simulink model "tqdtqr_rebuild_V3"  (R2021b)
settings: Solver=VariableStepAuto  StartTime=0.0  StopTime=10.0  RelTol=1e-3
undefined symbols (not defined in the file): ATQD_AfterTqMinGain_X_Deg, ATQD_APSCreepBaseTqD_X_kph, ATQD_APSCreepBaseTqD_Y_Deg, ATQD_APSCreepBaseTqR_X_kph, ATQD_APSCreepBaseTqR_Y_Deg, ATQD_APSCreepIterm_X_kph, ATQD_APSCreepIterm_Y_kph, ATQD_APSCreepPterm_X_kph, ATQD_APSCreepPterm_Y_kph, ATQD_APSDecReq_X_kph, ATQD_APSDecReq_Y_mps2, ATQD_APSDecReqCMD_X_kph, ATQD_APSDecReqTs_X_pct, ATQD_APSDecTimeGain_X_Deg, ATQD_APSDecTimeGain_Y_s, ATQD_APSReqLowSpd_X_Deg, ATQD_AutoHoldReleaseBPS_X_Deg, ATQD_AWDLoadTrqnsGain_X_kg, ATQD_AWDLoadTrqnsGain_Y_pct, ATQD_BOSEnBPSPosn_X_kph, ATQD_BOSMap_X_rpm, ATQD_BOSMap_Y_pct, ATQD_CreepBaseTqD_X_kph, ATQD_CreepBaseTqD_Y_Deg, ATQD_CreepBaseTqR_X_kph, ATQD_CreepBaseTqR_Y_Deg, ATQD_CreepBPSDisPosn_X_Deg, ATQD_CreepBPSDisPosnR_X_Deg, ATQD_CreepBPSEnPosn_X_Deg, ATQD_CreepBPSEnPosnR_X_Deg, ATQD_CreepDeltaTq_X_kph, ATQD_CreepIterm_X_kph, ATQD_CreepIterm_Y_kph, ATQD_CreepItermMaxLimit_X_pct, ATQD_CreepPreloadTime_X_kph, ATQD_CreepPreloadTq_X_kph, ATQD_CreepPreloadTq_Y_s, ATQD_CreepProtTq_X_Deg, ATQD_CreepPterm_X_kph, ATQD_CreepPterm_Y_kph, ATQD_CreepRrTqSpRat_X_rpm, ATQD_CreepRrTqSpRat_Y_Nm, ATQD_CreepTargetSpdD_X_pct, ATQD_CreepTargetSpdR_X_pct, ATQD_CreepUpLimitTq_X_rpm, ATQD_DecIneOPDHoldEnDelay_X_Deg, ATQD_DecIneOPDHoldEnDelay_Y_bar, ATQD_ECOTqMapD_X_rpm, ATQD_ECOTqMapD_Y_pct, ATQD_EMTqMapD_X_rpm, ATQD_EMTqMapD_Y_pct, ATQD_EOPDTqMapDCon_X_rpm, ATQD_EOPDTqMapDCon_Y_Deg, ATQD_EstInitVehWeight_X_c, ATQD_FAfterTqCMDGain_X_rpm, ATQD_FAfterTqCMDGain_Y_pct, ATQD_ForceLowSpd_X_Deg, ATQD_ForcePLimitSpd_X_Deg, ATQD_FrLossMAPLowV_X_rpm, ATQD_FrLossMAPLowV_Y_Nm ... (+949)
libraries: simulink x235, hcu_lib x208, tqr x63, tqd x6
(part 6 of 37)

== system tqdtqr_rebuild_V3/Output_Convert/CrashDetect ==
  BSCPIn_outputs : Inport
  Add1 : Sum
  Add2 : Sum
  Add3 : Sum
  Bus Selector : BusSelector  OutputSignals=VPMM_PowerSta_enum,VINP_CrashSignalGPIO_flg,VINP_CrashOutputSts_enum,task_time_s,VINP_FlashCrashDetd_flg,VINP_FlashCrashUnlockReq_flg,VBCM_CTDCtrl_enum,VBCM_CrashUnlkSuccess_flg
  Constant : Constant  Value=TRUE
  Constant1 : Constant  Value=ENUM_POWERSTA_ON
  Constant{3,8,10,19,23,36} (6 alike) : Constant  Value=KTQD_CrashPWMCnt_cnt
  Constant{6,11,20,26,31,34} (6 alike) : Constant  Value=ZERO_INT
  Constant12 : Constant  Value=KTQD_50MS_cnt
  Constant13 : Constant  Value=KTQD_PwrStaTimerforCrash_s
  Constant14 : Constant  Value=ENUM_CRASHSTATE_NOCRASH
  Constant15 : Constant  Value=KTQD_DiagHCrashTimer_s
  Constant16 : Constant  Value=ENUM_CRASHSTATE_NOCRASH
  Constant17 : Constant  Value=ENUM_CRASHSTATE_NOCRASH
  Constant18 : Constant  Value=KTQD_PwrStaTimerforCrash_s
  Constant2 : Constant  Value=ENUM_POWERSTA_READY
  Constant21 : Constant  Value=KTQD_50MS_cnt
  Constant22 : Constant  Value=ZERO_FLOAT
  Constant24 : Constant  Value=KTQD_NoDiagHCrashTimer_s
  Constant25 : Constant  Value=KTQD_DiagHCrashTimer_s
  Constant27 : Constant  Value=KTQD_190MS_cnt
  Constant28 : Constant  Value=KTQD_30MS_cnt
  Constant29 : Constant  Value=KTQD_50MS_cnt
  Constant30 : Constant  Value=KTQD_210MS_cnt
  Constant32 : Constant  Value=KTQD_NoDiagHCrashTimer_s
  Constant33 : Constant  Value=KTQD_PwrDownTimerforCrash_s
  Constant35 : Constant  Value=KTQD_210MS_cnt
  Constant37 : Constant  Value=KTQD_PwrDownTimerforCrash_s
  Constant38 : Constant  Value=TRUE
  Constant39 : Constant  Value=ENUM_CTDCTRL_UNLOCKALL
  Constant4 : Constant  Value=ONE_INT
  Constant{9,40..42} (4 alike) : Constant  Value=FALSE
  Constant43 : Constant  Value=KTQD_CrashDetdHoldTime_s
  Constant5 : Constant  Value=ENUM_POWERSTA_OFF
  Constant7 : Constant  Value=KTQD_210MS_cnt
  Data Type Conversion1 : DataTypeConversion
  Data Type Conversion2 : DataTypeConversion
  Detect Change : simulink/Logic and Bit Operations/Detect Change  vinit=0  OutDataTypeStr=boolean
  Detect Increase : simulink/Logic and Bit Operations/Detect Increase  vinit=0.0  OutDataTypeStr=boolean
  Equal : RelationalOperator  Operator=~=  OutDataTypeStr=boolean  RndMeth=Simplest
  Equal{1..2,6,10} (4 alike) : RelationalOperator  Operator===  OutDataTypeStr=boolean  RndMeth=Simplest
  Equal{3,7,9,11,13..14} (6 alike) : RelationalOperator  OutDataTypeStr=boolean  RndMeth=Simplest
  Equal12 : RelationalOperator  Operator=<  OutDataTypeStr=boolean  RndMeth=Simplest
  Equal4 : RelationalOperator  Operator=~=  OutDataTypeStr=boolean  RndMeth=Simplest
  Equal5 : RelationalOperator  Operator=<  OutDataTypeStr=boolean  RndMeth=Simplest
  Equal8 : RelationalOperator  Operator=~=  OutDataTypeStr=boolean  RndMeth=Simplest
  Hold : hcu_lib/Basic_Blocks/Hold  SystemSampleTime=-1  VariantActivationTime=update diagram  Latency=0  AutoFrameSizeCalculation=off
  Latch : hcu_lib/Basic_Blocks/Latch
  Latch2 : hcu_lib/Basic_Blocks/Latch
  Logical Operator{,9..10,13,16,21,23,26} (8 alike) : Logic  Operator=OR  AllPortsSameDT=off  OutDataTypeStr=boolean
  Logical Operator{1,3,7..8,18,20} (6 alike) : Logic  Operator=NOT  AllPortsSameDT=off  OutDataTypeStr=boolean
  Logical Operator{4..5,11..12,14..15,17,19,22} (9 alike) : Logic  AllPortsSameDT=off  OutDataTypeStr=boolean
  Logical Operator2 : Logic  Inputs=3  AllPortsSameDT=off  OutDataTypeStr=boolean
  Logical Operator6 : Logic  Inputs=3  AllPortsSameDT=off  OutDataTypeStr=boolean
  Relational Operator{,5..7,9} (5 alike) : RelationalOperator  Operator=>  OutDataTypeStr=boolean  RndMeth=Simplest
  Relational Operator1 : RelationalOperator  OutDataTypeStr=boolean  RndMeth=Simplest
  Relational Operator10 : RelationalOperator  Operator=<  OutDataTypeStr=boolean  RndMeth=Simplest
  Relational Operator2 : RelationalOperator  Operator=<=  OutDataTypeStr=boolean  RndMeth=Simplest
  Relational Operator3 : RelationalOperator  OutDataTypeStr=boolean  RndMeth=Simplest
  Relational Operator4 : RelationalOperator  Operator=<=  OutDataTypeStr=boolean  RndMeth=Simplest
  Relational Operator8 : RelationalOperator  Operator=<  OutDataTypeStr=boolean  RndMeth=Simplest
  SR_Latch : hcu_lib/Basic_Blocks/SR_Latch
  SR_Latch1 : hcu_lib/Basic_Blocks/SR_Latch
  Switch{,1,10..14} (7 alike) : Switch  Criteria=u2 ~= 0
  Switch{2..9} (8 alike) : Switch  Criteria=u2 > Threshold
  Timer{1..4} (4 alike) : hcu_lib/Basic_Blocks/Timer
  Unit Delay{,1..7} (8 alike) : UnitDelay  SampleTime=-1  HasFrameUpgradeWarning=on
  VTQD_CrashDetd_flg : Outport
  VTQD_DiagHCrash_flg : Outport  Port=2
  VTQD_CrashUnlockReq_flg : Outport  Port=3
  VTQD_CTDCtrl_enum : Outport  Port=4
  wires:
  Latch2/1 -> Switch14/2
  [VTQD_CrashStaRst_flg] -> SR_Latch1/2
  SR_Latch1/1 -> [VTQD_CrashDetdFromAPP_flg]  "VTQD_CrashDetdFromAPP_flg"
  [VTQD_CrashDetd_flg] -> Detect Increase/1
  Detect Increase/1 -> Hold/3
  Hold/1 -> Switch11/2
  [task_time_s] -> Hold/1
  Constant43/1 -> Hold/2
  Constant39/1 -> Switch11/1
  Switch11/1 -> VTQD_CTDCtrl_enum/1  "VTQD_CTDCtrl_enum"
  [VBCM_CTDCtrl_enum] -> Switch11/3
  Constant42/1 -> Switch14/1
  Constant41/1 -> Switch13/1
  Logical Operator26/1 -> Switch12/3
  Switch14/1 -> Logical Operator26/2
  [VTQD_CrashStaRst_flg] -> Latch2/1
  Constant40/1 -> Switch12/1
  [VTQD_CrashDetdFromAPP_flg] -> Logical Operator26/1
  [VBCM_CrashUnlkSuccess_flg] -> Switch12/2
  [VTQD_FlashCrashUnlockReq_flg] -> Switch14/3
  Switch12/1 -> VTQD_CrashUnlockReq_flg/1, [VTQD_CrashUnlockReq_flg]  "VTQD_CrashUnlockReq_flg"
  Constant38/1 -> Unit Delay6/1
  Unit Delay6/1 -> Switch10/2
  Switch10/1 -> [VTQD_FlashCrashUnlockReq_flg], Unit Delay7/1
  Unit Delay7/1 -> Switch10/1
  [VINP_FlashCrashUnlockReq_flg] -> Switch10/3
  Unit Delay4/1 -> Switch/1
  Switch/1 -> [VTQD_FlashCrashUnlock_flg], Unit Delay4/1
  Constant/1 -> Unit Delay/1
  Unit Delay/1 -> Switch/2
  [VINP_FlashCrashDetd_flg] -> Switch/3
  Switch13/1 -> Logical Operator23/2
  [VTQD_CrashDetdFromAPP_flg] -> Logical Operator23/1
  Logical Operator23/1 -> VTQD_CrashDetd_flg/1, [VTQD_CrashDetd_flg]  "VTQD_CrashDetd_flg"
  [VTQD_CrashStaRst_flg] -> Latch/1
  Latch/1 -> Switch13/2
  [VTQD_FlashCrashUnlock_flg] -> Switch13/3
  [VTQD_PwrONorREADY_flg] -> Detect Change/1, Logical Operator22/2
  Logical Operator/1 -> [VTQD_PwrONorREADY_flg]
  Detect Change/1 -> Logical Operator22/1
  Constant37/1 -> Equal14/2
  Equal2/1 -> Logical Operator/2
  Constant1/1 -> Equal1/2
  [task_time_s] -> Timer1/3
  Constant2/1 -> Equal2/2
  [VPMM_PowerSta_enum] -> Equal1/1
  Constant13/1 -> Equal7/2
  Timer2/1 -> Equal7/1
  Equal14/1 -> Timer2/2  "VTQD_PwrDownTimerReady_flg"
  Timer1/1 -> Equal14/1
  Logical Operator22/1 -> [VTQD_CrashStaRst_flg]
  Constant33/1 -> Timer1/4
  [task_time_s] -> Timer2/3
  [VTQD_PwrONorREADY_flg] -> Logical Operator3/1, Timer1/2, Timer2/1
  Constant18/1 -> Timer2/4
  Equal7/1 -> [VTQD_PwrStaTimerReady_flg]  "VTQD_PwrStaTimerReady_flg"
  Equal1/1 -> Logical Operator/1
  Logical Operator3/1 -> Timer1/1
  [VPMM_PowerSta_enum] -> Equal2/1
  Data Type Conversion1/1 -> Add3/2
  Constant8/1 -> Relational Operator8/2
  Relational Operator8/1 -> Data Type Conversion1/1
  [VTQD_CrashCountEN_flg] -> Switch6/2
  [VTQD_PwrStaTimerReady_flg] -> Switch7/2
  Constant29/1 -> Relational Operator2/2
  Unit Delay3/1 -> Equal/1
  Constant26/1 -> Switch7/3
  Switch6/1 -> Switch3/1
  Logical Operator10/1 -> [VTQD_CrashCountEN_flg]
  Constant22/1 -> Relational Operator/2
  Add2/1 -> Switch2/3
  [VTQD_CrashChange_flg] -> Switch3/2
  Logical Operator6/1 -> Logical Operator10/2
  Constant28/1 -> Relational Operator1/2
  Logical Operator2/1 -> Logical Operator10/1
  Switch3/1 -> Switch7/1
  Equal/1 -> [VTQD_CrashChange_flg]
  Add3/1 -> Switch6/1
  Relational Operator3/1 -> Logical Operator6/2
  Constant6/1 -> Switch6/3
  Constant4/1 -> Add2/2
  Relational Operator2/1 -> Logical Operator2/3
  Logical Operator1/1 -> Logical Operator2/1
  [VTQD_fCrash_cnt] -> Relational Operator8/1, Add3/1
  Switch2/1 -> Unit Delay1/1
  Unit Delay5/1 -> [VTQD_fCrash_cnt], Equal3/1  "VTQD_fCrash_cnt"
  Relational Operator/1 -> Equal/2, Unit Delay3/1
  [VTQD_CrashChange_flg] -> Switch2/2
  [VINP_CrashSignalGPIO_flg] -> Logical Operator1/1
  [VTQD_CrashCount_enum] -> Relational Operator2/1, Relational Operator1/1
  Relational Operator1/1 -> Logical Operator2/2
  Constant31/1 -> Switch2/1
  [VINP_CrashSignalGPIO_flg] -> Relational Operator/1
  Constant10/1 -> Equal3/2
  [VTQD_PwrStaTimerReady_flg] -> Logical Operator12/2
  Logical Operator12/1 -> Logical Operator13/2, [VTQD_CrashOutputSts_flg]
  Equal4/1 -> Logical Operator12/1
  Constant14/1 -> Equal4/2
  [VINP_CrashOutputSts_enum] -> Equal4/1
  Switch7/1 -> Unit Delay5/1
  Unit Delay1/1 -> [VTQD_CrashCount_enum]
  [VTQD_CrashCount_enum] -> Add2/1
  Logical Operator4/1 -> Logical Operator9/2
  [VTQD_CrashCount_enum] -> Relational Operator6/1
  Relational Operator6/1 -> Logical Operator4/2
  [VINP_CrashSignalGPIO_flg] -> Logical Operator8/1
  Logical Operator5/1 -> Logical Operator9/1
  Constant7/1 -> Relational Operator6/2
  Constant11/1 -> Switch4/1
  Logical Operator8/1 -> Logical Operator4/1
  [VTQD_fCrash_cnt] -> Switch4/3
  [VTQD_CrashCount_enum] -> Relational Operator7/1
  Logical Operator9/1 -> Switch4/2
  Relational Operator7/1 -> Logical Operator5/2
  [VINP_CrashSignalGPIO_flg] -> Logical Operator5/1
  Constant12/1 -> Relational Operator7/2
  Switch4/1 -> Switch3/3
  Equal3/1 -> Logical Operator13/1
  Logical Operator13/1 -> SR_Latch1/1
  [VINP_CrashSignalGPIO_flg] -> Logical Operator6/1
  Relational Operator4/1 -> Logical Operator6/3
  Constant30/1 -> Relational Operator4/2
  Constant27/1 -> Relational Operator3/2
  [VTQD_CrashCount_enum] -> Relational Operator4/1, Relational Operator3/1
  [VINP_CrashSignalGPIO_flg] -> Logical Operator19/1
  Equal12/1 -> Logical Operator17/1
  Unit Delay2/1 -> Equal9/1, Equal12/1, [test_crash_cnt]
  Equal9/1 -> Logical Operator14/1
  [VINP_CrashOutputSts_enum] -> Equal8/1
  Data Type Conversion2/1 -> Add1/2
  [VTQD_CrashChange_flg] -> Switch5/2
  [test_crash_cnt] -> Relational Operator10/1, Add1/1
  Switch9/1 -> Switch5/1
  Logical Operator21/1 -> Switch8/2
  Constant15/1 -> Equal11/2
  Relational Operator5/1 -> Logical Operator15/2
  Equal6/1 -> Switch1/2
  Relational Operator10/1 -> Data Type Conversion2/1
  Constant34/1 -> Switch9/3
  [task_time_s] -> Timer4/3
  Logical Operator17/1 -> Logical Operator16/2
  Constant36/1 -> Relational Operator10/2
  SR_Latch/1 -> VTQD_DiagHCrash_flg/1  "VTQD_DiagHCrash_flg"
  Equal10/1 -> Logical Operator17/2
  Logical Operator20/1 -> Logical Operator15/1
  Constant20/1 -> Switch8/1
  Equal13/1 -> Switch1/3
  Relational Operator9/1 -> Logical Operator19/2
  Constant16/1 -> Equal8/2
  [VTQD_CrashCount_enum] -> Relational Operator9/1
  [VINP_CrashOutputSts_enum] -> Equal10/1
  Switch8/1 -> Switch5/3
  Equal11/1 -> Logical Operator11/2
  Logical Operator19/1 -> Logical Operator21/1
  Constant19/1 -> Equal9/2
  Constant21/1 -> Relational Operator9/2
  Constant17/1 -> Equal10/2
  Logical Operator18/1 -> Timer4/2
  [test_crash_cnt] -> Switch8/3
  Constant3/1 -> Equal5/2
  Logical Operator15/1 -> Logical Operator21/2
  Constant35/1 -> Relational Operator5/2
  Constant32/1 -> Timer4/4
  [VTQD_CrashCountEN_flg] -> Switch9/2
  Constant23/1 -> Equal12/2
  Equal8/1 -> Logical Operator14/2
  Constant24/1 -> Equal13/2
  [VPMM_PowerSta_enum] -> Equal6/1
  Add1/1 -> Switch9/1
  Logical Operator11/1 -> SR_Latch/1
  [VTQD_CrashOutputSts_flg] -> Logical Operator7/1, Timer3/1
  Switch1/1 -> SR_Latch/2
  Timer4/1 -> Equal13/1
  Constant9/1 -> Switch1/1
  [VINP_CrashSignalGPIO_flg] -> Logical Operator20/1
  [VTQD_fCrash_cnt] -> Equal5/1
  Logical Operator7/1 -> Timer3/2
  Switch5/1 -> Unit Delay2/1
  Equal5/1 -> Logical Operator11/1
  [task_time_s] -> Timer3/3
  Constant5/1 -> Equal6/2
  [VTQD_CrashCount_enum] -> Relational Operator5/1
  Constant25/1 -> Timer3/4
  Logical Operator16/1 -> Logical Operator18/1, Timer4/1
  Timer3/1 -> Equal11/1
  Logical Operator14/1 -> Logical Operator16/1
  BSCPIn_outputs/1 -> Bus Selector/1
  Bus Selector/1 -> [VPMM_PowerSta_enum]  "<VPMM_PowerSta_enum>"
  Bus Selector/2 -> [VINP_CrashSignalGPIO_flg]  "<VINP_CrashSignalGPIO_flg>"
  Bus Selector/3 -> [VINP_CrashOutputSts_enum]  "<VINP_CrashOutputSts_enum>"
  Bus Selector/4 -> [task_time_s]  "<task_time_s>"
  Bus Selector/5 -> [VINP_FlashCrashDetd_flg]  "<VINP_FlashCrashDetd_flg>"
  Bus Selector/6 -> [VINP_FlashCrashUnlockReq_flg]  "<VINP_FlashCrashUnlockReq_flg>"
  Bus Selector/7 -> [VBCM_CTDCtrl_enum]  "<VBCM_CTDCtrl_enum>"
  Bus Selector/8 -> [VBCM_CrashUnlkSuccess_flg]  "<VBCM_CrashUnlkSuccess_flg>"

== system tqdtqr_rebuild_V3/Output_Convert/ESC//TCS demand torque ==
  note: Calculate Fr/Rr ESC/TCS demand torque
  BSCPIn_outputs : Inport
  BInpConvert_outputs : Inport  Port=2
  BMain_outputs : Inport  Port=3
  AND6 : Logic  AllPortsSameDT=off  OutDataTypeStr=boolean
  AND7 : Logic  AllPortsSameDT=off  OutDataTypeStr=boolean
  Bus Selector : BusSelector  OutputSignals=task_time_s
  Bus Selector1 : BusSelector  OutputSignals=VTQD_CreepBaseTqD_Nm,VTQD_FrEDUSpRat_rat,VTQD_CreepTCSActive_flg,VTQD_RrEDUSpRat_rat,VTQD_WhlTqCapMotFr_Nm,VTQD_WhlTqCapGenFr_Nm,VTQR_FrFirstOrderInpTs_c,VTQR_FrRateLimitInc_Nm,VTQR_FrRateLimitDec_Nm,VTQD_WhlTqCapMotRr_Nm,VTQD_WhlTqCapGenRr_Nm,VTQR_RrFirstOrderInpTs_c,VTQR_RrRateLimitInc_Nm,VTQR_RrRateLimitDec_Nm
  Bus Selector2 : BusSelector  OutputSignals=VTQD_CoordTqDem_Nm,VTQD_CoordTqDemRr_Nm
  Constant23 : Constant  Value=ZERO_FLOAT
  Constant24 : Constant  Value=ZERO_FLOAT
  Constant25 : Constant  Value=KTQD_TCSCreepDriveTqSW_flg  VectorParams1D=off  SampleTime=-1
  Constant26 : Constant  Value=KTQD_TCSCreepDriveTqSW_flg  VectorParams1D=off  SampleTime=-1
  FirstOrderFilter1 : hcu_lib/Basic_Blocks/FirstOrderFilter
  FirstOrderFilter2 : hcu_lib/Basic_Blocks/FirstOrderFilter
  Product2 : Product
  Product3 : Product
  RateLimit1 : tqr/TQR/Determine Torque Request/TorqueArbitrament/TorqueSmooth/RateLimit
  RateLimit2 : tqr/TQR/Determine Torque Request/TorqueArbitrament/TorqueSmooth/RateLimit
  Saturation Dynamic1 : simulink/Discontinuities/Saturation Dynamic  OutMin=[]  OutMax=[]  OutDataTypeStr=Inherit: Same as second input  OutDataType=fixdt(1, 16)  OutScaling=2^-10  DoSatur=off
  Saturation Dynamic2 : simulink/Discontinuities/Saturation Dynamic  OutMin=[]  OutMax=[]  OutDataTypeStr=Inherit: Same as second input  OutDataType=fixdt(1, 16)  OutScaling=2^-10  DoSatur=off
  Switch6 : Switch  Criteria=u2 ~= 0
      settings: AttributesFormatString=%<Criteria>
  Switch7 : Switch  Criteria=u2 ~= 0
      settings: AttributesFormatString=%<Criteria>
  VTQD_DriverWhlTqDemFr_Nm : Outport
  VTQD_DriverWhlTqDemRr_Nm : Outport  Port=2
  wires:
  BSCPIn_outputs/1 -> Bus Selector/1
  BInpConvert_outputs/1 -> Bus Selector1/1
  BMain_outputs/1 -> Bus Selector2/1
  Bus Selector/1 -> [task_time_s]  "<task_time_s>"
  Bus Selector2/1 -> [VTQD_CoordTqDemFr_Nm]  "<VTQD_CoordTqDem_Nm>"
  Bus Selector1/1 -> [VTQD_CreepBaseTqD_Nm]  "<VTQD_CreepBaseTqD_Nm>"
  Bus Selector1/2 -> [VTQD_FrEDUSpRat_rat]  "<VTQD_FrEDUSpRat_rat>"
  Bus Selector1/3 -> [VTQD_CreepTCSActive_flg]  "<VTQD_CreepTCSActive_flg>"
  Bus Selector1/4 -> [VTQD_RrEDUSpRat_rat]  "<VTQD_RrEDUSpRat_rat>"
  [task_time_s] -> FirstOrderFilter2/2
  Product3/1 -> Switch7/1
  [VTQD_WhlTqCapMotRr_Nm] -> Saturation Dynamic2/1
  [VTQD_CreepTCSActive_flg] -> AND7/1
  [VTQD_WhlTqCapGenRr_Nm] -> Saturation Dynamic2/3
  Switch7/1 -> [VTQD_DriverWhlTqDemRr_Nm]  "VTQD_DriverWhlTqDemRr_Nm"
  [VTQD_CoordTqDemFr_Nm] -> Saturation Dynamic1/2
  [task_time_s] -> FirstOrderFilter1/2
  Saturation Dynamic2/1 -> FirstOrderFilter1/1
  Constant26/1 -> AND7/2
  Constant23/1 -> RateLimit1/2
  [VTQD_WhlTqCapMotFr_Nm] -> Saturation Dynamic1/1
  [VTQD_CreepBaseTqD_Nm] -> Product2/1
  Saturation Dynamic1/1 -> FirstOrderFilter2/1
  FirstOrderFilter1/1 -> RateLimit1/1
  AND6/1 -> Switch6/2
  [task_time_s] -> RateLimit2/3
  Constant24/1 -> RateLimit2/2
  [VTQD_CreepTCSActive_flg] -> AND6/1
  [VTQR_RrFirstOrderInpTs_c] -> FirstOrderFilter1/3
  RateLimit1/1 -> Switch7/3
  Product2/1 -> Switch6/1
  [VTQD_CreepBaseTqD_Nm] -> Product3/1
  [VTQD_CoordTqDemRr_Nm] -> Saturation Dynamic2/2
  RateLimit2/1 -> Switch6/3
  FirstOrderFilter2/1 -> RateLimit2/1
  [VTQR_RrRateLimitDec_Nm] -> RateLimit1/5
  Constant25/1 -> AND6/2
  [VTQR_RrRateLimitInc_Nm] -> RateLimit1/4
  [VTQD_FrEDUSpRat_rat] -> Product2/2
  [VTQR_FrFirstOrderInpTs_c] -> FirstOrderFilter2/3
  [VTQD_WhlTqCapGenFr_Nm] -> Saturation Dynamic1/3
  [VTQD_RrEDUSpRat_rat] -> Product3/2
  Switch6/1 -> [VTQD_DriverWhlTqDemFr_Nm]  "VTQD_DriverWhlTqDemFr_Nm"
  [task_time_s] -> RateLimit1/3
  AND7/1 -> Switch7/2
  [VTQR_FrRateLimitDec_Nm] -> RateLimit2/5
  [VTQR_FrRateLimitInc_Nm] -> RateLimit2/4
  [VTQD_DriverWhlTqDemFr_Nm] -> VTQD_DriverWhlTqDemFr_Nm/1
  [VTQD_DriverWhlTqDemRr_Nm] -> VTQD_DriverWhlTqDemRr_Nm/1
  Bus Selector1/5 -> [VTQD_WhlTqCapMotFr_Nm]  "<VTQD_WhlTqCapMotFr_Nm>"
  Bus Selector1/6 -> [VTQD_WhlTqCapGenFr_Nm]  "<VTQD_WhlTqCapGenFr_Nm>"
  Bus Selector1/7 -> [VTQR_FrFirstOrderInpTs_c]  "<VTQR_FrFirstOrderInpTs_c>"
  Bus Selector1/8 -> [VTQR_FrRateLimitInc_Nm]  "<VTQR_FrRateLimitInc_Nm>"
  Bus Selector1/9 -> [VTQR_FrRateLimitDec_Nm]  "<VTQR_FrRateLimitDec_Nm>"
  Bus Selector1/10 -> [VTQD_WhlTqCapMotRr_Nm]  "<VTQD_WhlTqCapMotRr_Nm>"
  Bus Selector2/2 -> [VTQD_CoordTqDemRr_Nm]  "<VTQD_CoordTqDemRr_Nm>"
  Bus Selector1/11 -> [VTQD_WhlTqCapGenRr_Nm]  "<VTQD_WhlTqCapGenRr_Nm>"
  Bus Selector1/12 -> [VTQR_RrFirstOrderInpTs_c]  "<VTQR_RrFirstOrderInpTs_c>"
  Bus Selector1/13 -> [VTQR_RrRateLimitInc_Nm]  "<VTQR_RrRateLimitInc_Nm>"
  Bus Selector1/14 -> [VTQR_RrRateLimitDec_Nm]  "<VTQR_RrRateLimitDec_Nm>"

== system tqdtqr_rebuild_V3/Output_Convert/Equivalent Acceleration Pedal Switch signal ==
  note: Equivalent Acceleration Pedal Switch signal
  BSCPIn_outputs : Inport
  BInpConvert_outputs : Inport  Port=2
  BMain_outputs : Inport  Port=3
  AND1 : Logic  Operator=OR  AllPortsSameDT=off  OutDataTypeStr=boolean
  AND25 : Logic  Inputs=3  AllPortsSameDT=off  OutDataTypeStr=boolean
  Bus Selector : BusSelector  OutputSignals=task_time_s,VVMC_ADASWhlTqReq_Nm,VVMC_ACCRequiredAccel_mps2,VTQD_LowIdleAccPedal_flg,VVMC_ACCPedalOvrd_flg,VVMC_ADASActive_flg
  Bus Selector1 : BusSelector  OutputSignals=VTQD_VehActSpd_kph,VTQD_BrkSwSta_flg,VTQD_CreepTCSActive_flg
  Bus Selector2 : BusSelector  OutputSignals=VTQD_CoordTqDem_Nm
  Constant107 : Constant  Value=ONE_PERCENT
  Constant108 : Constant  Value=KTQD_EquivAccPedBaseTq_Nm
  Constant109 : Constant  Value=eps
  Constant145 : Constant  Value=FALSE
  Constant146 : Constant  Value=KTQD_EquivAccPedalDisSpd_kph
  Constant26 : Constant  Value=TRUE
  Constant45 : Constant  Value=FALSE
  Constant8 : Constant  Value=KTQD_ADASLowIdleWhlTq_Nm
  Constant85 : Constant  Value=KTQD_ACCReqCMdBond_mps2
  Constant93 : Constant  Value=KTQD_EquivAccPedalDelay_s
  Data Type Conversion6 : DataTypeConversion  OutDataTypeStr=single
  DelayEnable4 : hcu_lib/Basic_Blocks/DelayEnable
  Divide : Product  Inputs=*//
  KTQD_EquivAccPedEn_pct KTQD_EquivAccPedDis_pct : Relay  OnSwitchValue=KTQD_EquivAccPedEn_pct  OffSwitchValue=KTQD_EquivAccPedDis_pct  OutDataTypeStr=boolean
  KTQD_EquivAccPedUpLim_pct KTQD_EquivAccPedLowLim_pct : Saturate  UpperLimit=KTQD_EquivAccPedUpLim_pct  LowerLimit=KTQD_EquivAccPedLowLim_pct
  Logical Operator22 : Logic  Operator=NOT  AllPortsSameDT=off  OutDataTypeStr=boolean
  Max : MinMax  Function=max  Inputs=2
  OR6 : Logic  Operator=OR  AllPortsSameDT=off  OutDataTypeStr=boolean
  Relational Operator : RelationalOperator  OutDataTypeStr=boolean  RndMeth=Simplest
  Relational Operator5 : RelationalOperator  OutDataTypeStr=boolean  RndMeth=Simplest
  Relational Operator7 : RelationalOperator  Operator=<=  OutDataTypeStr=boolean  RndMeth=Simplest
  Switch{25..27,30} (4 alike) : Switch  Criteria=u2 ~= 0
      settings: AttributesFormatString=%<Criteria>
  VTQD_EquivAccPedalSWSta_flg : Outport
  wires:
  Constant108/1 -> Max/1
  [VTQD_CoordTqDem_Nm] -> Divide/1
  [VVMC_ACCPedalOvrd_flg] -> Switch26/2
  [VTQD_LowIdleAccPedal_flg] -> AND25/1
  Switch25/1 -> [VTQD_EquivAccPedalSWSta_flg]  "VTQD_EquivAccPedalSWSta_flg"
  Constant85/1 -> Relational Operator5/2
  Relational Operator7/1 -> AND25/2
  Relational Operator5/1 -> AND1/2
  Constant45/1 -> Switch27/3
  Constant8/1 -> Relational Operator/2
  [task_time_s] -> DelayEnable4/3
  AND25/1 -> Switch30/2
  Constant146/1 -> Relational Operator7/2
  Divide/1 -> KTQD_EquivAccPedUpLim_pct KTQD_EquivAccPedLowLim_pct/1
  Relational Operator/1 -> AND1/1
  Constant26/1 -> Switch27/1
  KTQD_EquivAccPedUpLim_pct KTQD_EquivAccPedLowLim_pct/1 -> KTQD_EquivAccPedEn_pct KTQD_EquivAccPedDis_pct/1  "VTQD_EquivAccPed_pct"
  Switch30/1 -> Switch25/3  "VTQD_EquivAccPed_flg"
  [VTQD_LowIdleAccPedal_flg] -> Logical Operator22/1
  Constant145/1 -> Switch30/1
  Logical Operator22/1 -> Switch26/1
  Switch27/1 -> Switch26/3
  OR6/1 -> Switch30/3
  [VTQD_VehActSpd_kph] -> Relational Operator7/1
  Max/1 -> Divide/2
  Data Type Conversion6/1 -> Max/2
  Constant93/1 -> DelayEnable4/2
  Switch26/1 -> Switch25/1
  AND1/1 -> DelayEnable4/1
  DelayEnable4/1 -> Switch27/2
  [VTQD_CreepTCSActive_flg] -> OR6/2
  Constant107/1 -> Divide/3
  KTQD_EquivAccPedEn_pct KTQD_EquivAccPedDis_pct/1 -> OR6/1
  Constant109/1 -> Data Type Conversion6/1
  [VVMC_ADASWhlTqReq_Nm] -> Relational Operator/1
  [VTQD_BrkSwSta_flg] -> AND25/3
  [VVMC_ADASActive_flg] -> Switch25/2
  [VVMC_ACCRequiredAccel_mps2] -> Relational Operator5/1
  [VTQD_EquivAccPedalSWSta_flg] -> VTQD_EquivAccPedalSWSta_flg/1
  BSCPIn_outputs/1 -> Bus Selector/1
  BInpConvert_outputs/1 -> Bus Selector1/1
  Bus Selector/1 -> [task_time_s]  "<task_time_s>"
  Bus Selector/2 -> [VVMC_ADASWhlTqReq_Nm]  "<VVMC_ADASWhlTqReq_Nm>"
  Bus Selector/3 -> [VVMC_ACCRequiredAccel_mps2]  "<VVMC_ACCRequiredAccel_mps2>"
  Bus Selector/4 -> [VTQD_LowIdleAccPedal_flg]  "<VTQD_LowIdleAccPedal_flg>"
  Bus Selector/5 -> [VVMC_ACCPedalOvrd_flg]  "<VVMC_ACCPedalOvrd_flg>"
  Bus Selector/6 -> [VVMC_ADASActive_flg]  "<VVMC_ADASActive_flg>"
  Bus Selector1/1 -> [VTQD_VehActSpd_kph]  "<VTQD_VehActSpd_kph>"
  Bus Selector1/2 -> [VTQD_BrkSwSta_flg]  "<VTQD_BrkSwSta_flg>"
  Bus Selector1/3 -> [VTQD_CreepTCSActive_flg]  "<VTQD_CreepTCSActive_flg>"
  BMain_outputs/1 -> Bus Selector2/1
  Bus Selector2/1 -> [VTQD_CoordTqDem_Nm]  "<VTQD_CoordTqDem_Nm>"

== system tqdtqr_rebuild_V3/Output_Convert/ExtTqFuncHandShaking ==
  BSCPIn_outputs : Inport
  Bus Selector : BusSelector  OutputSignals=VPMM_PowerSta_enum,VTQD_LimpHomeAct_flg,VDDM_EPBSigErrCFS_flg,VDDM_EPB1Err_flg,VINP_EPBErrSta_enum,VDDM_Shifter1Err_flg,VDDM_ShifterSigErrCFS_flg,VVMC_APSActive_flg,VINP_DrDoorSW_flg,VINP_PsDoorSW_flg,VINP_RRDoorSW_flg,VINP_RLDoorSW_flg,VINP_HoodSW_flg,VINP_TailgateSW_flg,VDDM_4D2CErr_flg
  Constant1 : Constant  Value=KTQD_ExtTqAllow_flg_ovrdflg
  Constant10 : Constant  Value=TRUE
  Constant11 : Constant  Value=FALSE
  Constant12 : Constant  Value=ENUM_EPBERROR_NORMAL
  Constant13 : Constant  Value=KTQD_ExtDoorAllow_flg_ovrdflg
  Constant14 : Constant  Value=KTQD_ExtDoorAllow_flg_ovrdval
  Constant15 : Constant  Value=ENUM_POWERSTA_READY
  Constant16 : Constant  Value=ENUM_POWERSTA_ON
  Constant17 : Constant  Value=ENUM_POWERSTA_READY
  Constant18 : Constant  Value=ENUM_POWERSTA_ON
  Constant19 : Constant  Value=KTQD_PassAPSActive_flg_ovrdflg
  Constant2 : Constant  Commented=on  Value=ENUM_DCDCFAULTSTA_WORKING
  Constant20 : Constant  Value=KTQD_PassAPSActive_flg_ovrdflg
  Constant21 : Constant  Value=KTQD_PassAPSActive_flg_ovrdval
  Constant22 : Constant  Value=KTQD_PassAPSActive_flg_ovrdval
  Constant3 : Constant  Value=KTQD_ExtTqAllow_flg_ovrdval
  Constant4 : Constant  Commented=on  Value=ENUM_DCDCFAULTSTA_WORKING
  Constant5 : Constant  Commented=on  Value=ENUM_EPBERROR_NORMAL
  Constant6 : Constant  Value=KTQD_ExtShftAllow_flg_ovrdflg
  Constant7 : Constant  Value=KTQD_ExtShftAllow_flg_ovrdval
  Constant8 : Constant  Value=TRUE
  Constant9 : Constant  Value=FALSE
  Equal1 : RelationalOperator  Commented=on  Operator===  OutDataTypeStr=boolean  RndMeth=Simplest
  Equal2 : RelationalOperator  Commented=on  Operator===  OutDataTypeStr=boolean  RndMeth=Simplest
  Equal3 : RelationalOperator  Commented=on  Operator===  OutDataTypeStr=boolean  RndMeth=Simplest
  Equal{4..8} (5 alike) : RelationalOperator  Operator===  OutDataTypeStr=boolean  RndMeth=Simplest
  From1 : From  Commented=on  GotoTag=VTQD_MCUReady4Ext_flg
  From2 : From  Commented=on  GotoTag=VINP_HVBattErr_flg
  From3 : From  Commented=on  GotoTag=VINP_DCDCFaultSta_enum
  From4 : From  Commented=on  GotoTag=VTQD_MCUReady4Ext_flg
  From5 : From  Commented=on  GotoTag=VINP_HVBattErr_flg
  From6 : From  Commented=on  GotoTag=VINP_DCDCFaultSta_enum
  From8 : From  Commented=on  GotoTag=VINP_EPBErrSta_enum
  LiuzgSwitch{1..7} (7 alike) : Switch  Criteria=u2 ~= 0
      settings: AttributesFormatString=<%<Criteria>>
  Logical Operator : Logic  Commented=on  Operator=NOT  AllPortsSameDT=off  OutDataTypeStr=boolean
  Logical Operator1 : Logic  Commented=on  Operator=NOT  AllPortsSameDT=off  OutDataTypeStr=boolean
  Logical Operator{4..7,9..10} (6 alike) : Logic  Operator=NOT  AllPortsSameDT=off  OutDataTypeStr=boolean
  Logical Operator11 : Logic  AllPortsSameDT=off  OutDataTypeStr=boolean
  Logical Operator12 : Logic  AllPortsSameDT=off  OutDataTypeStr=boolean
  Logical Operator2 : Logic  Operator=OR  AllPortsSameDT=off  OutDataTypeStr=boolean
  Logical Operator3 : Logic  Operator=OR  AllPortsSameDT=off  OutDataTypeStr=boolean
  Logical Operator8 : Logic  Inputs=3  AllPortsSameDT=off  OutDataTypeStr=boolean
  NOT{,1..6} (7 alike) : Logic  Operator=NOT  AllPortsSameDT=off  OutDataTypeStr=boolean
  OR : Logic  AllPortsSameDT=off  OutDataTypeStr=boolean
  OR1 : Logic  Inputs=5  AllPortsSameDT=off  OutDataTypeStr=boolean
  OR2 : Logic  Inputs=7  AllPortsSameDT=off  OutDataTypeStr=boolean
  VTQD_ExternalTqAllow_flg : Outport
  VTQD_ExtShftAllow_flg : Outport  Port=2
  VTQD_ExtDoorAllow_flg : Outport  Port=3
  wires:
  [VDDM_EPB1Err_flg] -> Logical Operator10/1
  Logical Operator9/1 -> Logical Operator8/1
  [VINP_HoodSW_flg] -> NOT4/1
  Constant15/1 -> Equal5/2
  Logical Operator5/1 -> OR1/5
  Constant13/1 -> LiuzgSwitch5/2
  NOT3/1 -> OR2/4
  Logical Operator8/1 -> OR1/2
  Equal5/1 -> Logical Operator2/1
  [VPMM_PwrSta_enum] -> Equal5/1
  Logical Operator11/1 -> LiuzgSwitch6/2
  Constant4/1 -> Equal1/2
  [VDDM_Shifter1Err_flg] -> Logical Operator4/1
  LiuzgSwitch7/1 -> LiuzgSwitch2/3
  Constant20/1 -> Logical Operator12/2
  NOT/1 -> OR2/1
  Constant12/1 -> Equal4/2
  [VINP_EPBErrSta_enum] -> Equal4/1
  From5/1 -> Logical Operator1/1
  Constant14/1 -> LiuzgSwitch5/1
  Constant9/1 -> LiuzgSwitch3/3
  Constant8/1 -> LiuzgSwitch3/1
  [VINP_DrDoorSW_flg] -> NOT/1
  LiuzgSwitch2/1 -> VTQD_ExtShftAllow_flg/1  "VTQD_ExtShftAllow_flg"
  Constant1/1 -> LiuzgSwitch1/2
  From2/1 -> Logical Operator/1
  From3/1 -> Equal2/1
  Constant3/1 -> LiuzgSwitch1/1
  Constant17/1 -> Equal7/2
  Equal8/1 -> Logical Operator3/2
  [VINP_RLDoorSW_flg] -> NOT3/1
  [VINP_PsDoorSW_flg] -> NOT1/1
  Constant11/1 -> LiuzgSwitch4/3
  NOT1/1 -> OR2/2
  Constant16/1 -> Equal6/2
  Constant2/1 -> Equal2/2
  NOT2/1 -> OR2/3
  OR2/1 -> LiuzgSwitch5/3
  NOT5/1 -> OR2/6
  NOT4/1 -> OR2/5
  LiuzgSwitch4/1 -> LiuzgSwitch6/3
  [VVMC_APSActive_flg] -> Logical Operator11/1
  Equal7/1 -> Logical Operator3/1
  Constant19/1 -> Logical Operator11/2
  [VPMM_PwrSta_enum] -> Equal7/1
  [VDDM_4D2CErr_flg] -> NOT6/1
  Constant10/1 -> LiuzgSwitch4/1
  OR1/1 -> LiuzgSwitch3/2
  Logical Operator4/1 -> OR1/4
  NOT6/1 -> OR2/7
  [VPMM_PwrSta_enum] -> Equal8/1
  Logical Operator12/1 -> LiuzgSwitch7/2
  LiuzgSwitch1/1 -> VTQD_ExternalTqAllow_flg/1  "VTQD_ExternalTqAllow_flg"
  [VTQD_LimpHomeAct_flg] -> Logical Operator7/1
  From6/1 -> Equal1/1
  LiuzgSwitch5/1 -> VTQD_ExtDoorAllow_flg/1  "VTQD_ExtDoorAllow_flg"
  [VVMC_APSActive_flg] -> Logical Operator12/1
  Constant21/1 -> LiuzgSwitch6/1
  LiuzgSwitch6/1 -> LiuzgSwitch1/3
  LiuzgSwitch3/1 -> LiuzgSwitch7/3
  Equal6/1 -> Logical Operator2/2
  [VDDM_ShifterSigErrCFS_flg] -> Logical Operator5/1
  Logical Operator7/1 -> OR1/3
  Constant5/1 -> Equal3/2
  Equal4/1 -> Logical Operator8/3
  Logical Operator2/1 -> OR1/1
  Constant22/1 -> LiuzgSwitch7/1
  From8/1 -> Equal3/1
  [VPMM_PwrSta_enum] -> Equal6/1
  [VTQD_LimpHomeAct_flg] -> Logical Operator6/1
  OR/1 -> LiuzgSwitch4/2
  [VDDM_EPBSigErrCFS_flg] -> Logical Operator9/1
  [VINP_TailgateSW_flg] -> NOT5/1
  Logical Operator3/1 -> OR/1
  Constant6/1 -> LiuzgSwitch2/2
  Constant7/1 -> LiuzgSwitch2/1
  Logical Operator10/1 -> Logical Operator8/2
  Logical Operator6/1 -> OR/2
  [VINP_RRDoorSW_flg] -> NOT2/1
  Constant18/1 -> Equal8/2
  BSCPIn_outputs/1 -> Bus Selector/1
  Bus Selector/1 -> [VPMM_PwrSta_enum]  "<VPMM_PowerSta_enum>"
  Bus Selector/2 -> [VTQD_LimpHomeAct_flg]  "<VTQD_LimpHomeAct_flg>"
  Bus Selector/3 -> [VDDM_EPBSigErrCFS_flg]  "<VDDM_EPBSigErrCFS_flg>"
  Bus Selector/4 -> [VDDM_EPB1Err_flg]  "<VDDM_EPB1Err_flg>"
  Bus Selector/5 -> [VINP_EPBErrSta_enum]  "<VINP_EPBErrSta_enum>"
  Bus Selector/6 -> [VDDM_Shifter1Err_flg]  "<VDDM_Shifter1Err_flg>"
  Bus Selector/7 -> [VDDM_ShifterSigErrCFS_flg]  "<VDDM_ShifterSigErrCFS_flg>"
  Bus Selector/8 -> [VVMC_APSActive_flg]  "<VVMC_APSActive_flg>"
  Bus Selector/9 -> [VINP_DrDoorSW_flg]  "<VINP_DrDoorSW_flg>"
  Bus Selector/10 -> [VINP_PsDoorSW_flg]  "<VINP_PsDoorSW_flg>"
  Bus Selector/11 -> [VINP_RRDoorSW_flg]  "<VINP_RRDoorSW_flg>"
  Bus Selector/12 -> [VINP_RLDoorSW_flg]  "<VINP_RLDoorSW_flg>"
  Bus Selector/13 -> [VINP_HoodSW_flg]  "<VINP_HoodSW_flg>"
  Bus Selector/14 -> [VINP_TailgateSW_flg]  "<VINP_TailgateSW_flg>"
  Bus Selector/15 -> [VDDM_4D2CErr_flg]  "<VDDM_4D2CErr_flg>"

== system tqdtqr_rebuild_V3/Output_Convert/P_Button_State_Judge ==
  BSCPIn_outputs : Inport
  BInpConvert_outputs : Inport  Port=2
  AND : Logic  Inputs=4  AllPortsSameDT=off  OutDataTypeStr=boolean
  Bus Selector : BusSelector  OutputSignals=VTQD_ShifterHandleCmd_enum,VVMC_APSActive_flg,VVMC_APSShiftPosnReq_enum,VINP_EPBSta_enum,VINP_VehSpeed_kph
  Bus Selector1 : BusSelector  OutputSignals=VTQD_ParkRequest_flg,VTQD_DOALatchReq_flg,VTQD_ForcePLimitSpd_kph
  Constant : Constant  Value=ENUM_EPBSTA_APPLIED
  Constant1 : Constant  Value=ENUM_PBUTTON_RELEASED
  Constant10 : Constant  Value=KTQD_DOAOPDReqSW_flg
  Constant11 : Constant  Value=KTQD_DOADisPButtonSpd_kph
  Constant12 : Constant  Value=ENUM_SHIFTCOMMAND_D
  Constant15 : Constant  Value=ENUM_SHIFTCOMMAND_N
  Constant2 : Constant  Value=ENUM_PBUTTON_PRESSED
  Constant3 : Constant  Value=ENUM_PBUTTON_INVALID
  Constant4 : Constant  Value=ENUM_SHIFTCOMMAND_NONE
  Constant5 : Constant  Value=ENUM_SHIFTCOMMAND_P
  Constant6 : Constant  Value=ENUM_PBUTTON_PRESSED
  Constant7 : Constant  Value=ENUM_SHIFTCOMMAND_P
  Constant8 : Constant  Value=ENUM_SHIFTCOMMAND_R
  Constant9 : Constant  Value=ENUM_EPBSTA_APPLIED
  Detect Decrease : simulink/Logic and Bit Operations/Detect Decrease  vinit=0.0  OutDataTypeStr=boolean
  Detect Decrease1 : simulink/Logic and Bit Operations/Detect Decrease  vinit=0.0  OutDataTypeStr=boolean
  Detect Increase : simulink/Logic and Bit Operations/Detect Increase  vinit=0.0  OutDataTypeStr=boolean
  Detect Increase1 : simulink/Logic and Bit Operations/Detect Increase  vinit=0.0  OutDataTypeStr=boolean
  Equal{,1..7} (8 alike) : RelationalOperator  Operator===  OutDataTypeStr=boolean  RndMeth=Simplest
  Logical Operator : Logic  Operator=OR  Inputs=4  AllPortsSameDT=off  OutDataTypeStr=boolean
  Logical Operator1 : Logic  Operator=OR  Inputs=3  AllPortsSameDT=off  OutDataTypeStr=boolean
  Logical Operator2 : Logic  Operator=OR  AllPortsSameDT=off  OutDataTypeStr=boolean
  Logical Operator3 : Logic  AllPortsSameDT=off  OutDataTypeStr=boolean
  Logical Operator4 : Logic  Operator=OR  Inputs=3  AllPortsSameDT=off  OutDataTypeStr=boolean
  NOT : Logic  Operator=NOT  AllPortsSameDT=off  OutDataTypeStr=boolean
  NOT1 : Logic  Operator=NOT  AllPortsSameDT=off  OutDataTypeStr=boolean
  Relational Operator : RelationalOperator  Operator=>  OutDataTypeStr=boolean  RndMeth=Simplest
  Relational Operator1 : RelationalOperator  Operator=<=  OutDataTypeStr=boolean  RndMeth=Simplest
  SR_Latch : hcu_lib/Basic_Blocks/SR_Latch
  SR_Latch1 : hcu_lib/Basic_Blocks/SR_Latch
  Switch1 : Switch  Criteria=u2 ~= 0
      settings: AttributesFormatString=%<Criteria>
  Switch2 : Switch  Criteria=u2 ~= 0
      settings: AttributesFormatString=%<Criteria>
  Switch4 : Switch  Criteria=u2 ~= 0
      settings: AttributesFormatString=%<Criteria>
  VTQD_PButtonSta_enum : Outport
  wires:
  Equal/1 -> [P]
  Constant12/1 -> Equal2/2
  [VTQD_ShifterHandleCmd_enum] -> Equal1/1
  Constant8/1 -> Equal1/2
  [VTQD_ShifterHandleCmd_enum] -> Equal/1
  Equal2/1 -> Logical Operator/3
  Constant15/1 -> Equal3/2
  Equal3/1 -> Logical Operator/2
  Equal1/1 -> Logical Operator/1
  Constant5/1 -> Equal/2
  [VTQD_ShifterHandleCmd_enum] -> Equal3/1
  [VTQD_ShifterHandleCmd_enum] -> Equal2/1
  Logical Operator/1 -> [RND]
  [VTQD_ShifterHandleCmd_enum] -> Equal4/1
  Constant4/1 -> Equal4/2
  Equal4/1 -> Logical Operator/4
  BSCPIn_outputs/1 -> Bus Selector/1
  BInpConvert_outputs/1 -> Bus Selector1/1
  Bus Selector/1 -> [VTQD_ShifterHandleCmd_enum]  "<VTQD_ShifterHandleCmd_enum>"
  Bus Selector/2 -> [VVMC_APSActive_flg]  "<VVMC_APSActive_flg>"
  Bus Selector/3 -> [VVMC_APSShiftPosnReq_enum]  "<VVMC_APSShiftPosnReq_enum>"
  Bus Selector/4 -> [VINP_EPBSta_enum]  "<VINP_EPBSta_enum>"
  Bus Selector1/1 -> [VTQD_ParkRequest_flg]  "<VTQD_ParkRequest_flg>"
  Logical Operator2/1 -> SR_Latch/2
  SR_Latch/1 -> Logical Operator1/1
  Detect Increase/1 -> SR_Latch/1
  Constant7/1 -> Equal6/2
  Constant3/1 -> Switch1/3
  Constant2/1 -> Switch1/1
  [VINP_VehSpeed_kph] -> Relational Operator1/1
  [P] -> Switch1/2
  Constant11/1 -> Relational Operator1/2
  Constant1/1 -> Switch4/1
  Logical Operator3/1 -> Detect Increase1/1, Detect Decrease1/1
  Relational Operator1/1 -> AND/4
  Constant10/1 -> NOT1/1
  Switch1/1 -> Switch4/3
  Relational Operator/1 -> AND/3
  [VTQD_ForcePLimitSpd_kph] -> Relational Operator/2
  Detect Decrease/1 -> Logical Operator2/1
  [VINP_EPBSta_enum] -> Equal5/1
  [VVMC_APSActive_flg] -> Logical Operator3/1
  Equal5/1 -> Logical Operator2/2
  Constant6/1 -> Switch2/1
  [RND] -> Switch4/2
  [VVMC_APSShiftPosnReq_enum] -> Equal6/1
  Constant9/1 -> Equal7/2
  AND/1 -> Logical Operator1/2
  [VTQD_DOALatchReq_flg] -> AND/1
  Detect Decrease1/1 -> Logical Operator4/1
  [VTQD_ParkRequest_flg] -> Detect Decrease/1, Detect Increase/1
  Constant/1 -> Equal5/2
  Logical Operator4/1 -> SR_Latch1/2
  Equal6/1 -> Logical Operator3/2
  Logical Operator1/1 -> Switch2/2
  [VINP_EPBSta_enum] -> Equal7/1
  Switch2/1 -> VTQD_PButtonSta_enum/1  "VTQD_PButtonSta_enum"
  NOT1/1 -> AND/2
  [VVMC_APSActive_flg] -> NOT/1
  [VINP_VehSpeed_kph] -> Relational Operator/1
  NOT/1 -> Logical Operator4/2
  Equal7/1 -> Logical Operator4/3
  SR_Latch1/1 -> Logical Operator1/3
  Switch4/1 -> Switch2/3
  Detect Increase1/1 -> SR_Latch1/1
  Bus Selector/5 -> [VINP_VehSpeed_kph]  "<VINP_VehSpeed_kph>"
  Bus Selector1/2 -> [VTQD_DOALatchReq_flg]  "<VTQD_DOALatchReq_flg>"
  Bus Selector1/3 -> [VTQD_ForcePLimitSpd_kph]  "<VTQD_ForcePLimitSpd_kph>"

== system tqdtqr_rebuild_V3/Output_Convert/Regen Limited Indicator signal ==
  note: Regen Limited Indicator signal
  BSCPIn_outputs : Inport
  BInpConvert_outputs : Inport  Port=2
  BMain_outputs : Inport  Port=3
  AND15 : Logic  AllPortsSameDT=off  OutDataTypeStr=boolean
  AND6 : Logic  Operator=OR  AllPortsSameDT=off  OutDataTypeStr=boolean
  AND8 : Logic  Operator=OR  AllPortsSameDT=off  OutDataTypeStr=boolean
  Bus Selector : BusSelector  OutputSignals=task_time_s,VTQD_RDCActive_enum,VINP_HVBattSOCDis_pct,VINP_HVBMTempMin_C,VINP_HVBMTempMax_C,VPMM_DrivetrainSelect_enum
  Bus Selector1 : BusSelector  OutputSignals=VTQD_GearActualPosn_enum,VTQD_WhlTqCapGenFr_Nm
  Bus Selector2 : BusSelector  OutputSignals=VTQD_CoordWhlTqDemFr_Nm,VTQD_CoordWhlTqDemRr_Nm
  Constant103 : Constant  Value=KTQD_RegenLimHVTempMin_C
  Constant104 : Constant  Value=KTQD_RegenLimHVTempMax_C
  Constant105 : Constant  Value=ENUM_RDCACTSTA_NOREQUEST
  Constant106 : Constant  Value=KTQD_RegenLimIndSOC_pct
  Constant126 : Constant  Value=KTQD_RgnLimIndStaDelay_s
  Constant91 : Constant  Value=ENUM_GEARACTUALPOSN_N
  Constant92 : Constant  Value=ENUM_GEARACTUALPOSN_P
  Constant94 : Constant  Value=ENUM_DRIVETRAIN_RWD
  Constant95 : Constant  Value=ENUM_DRIVETRAIN_FWD
  Delay17 : Delay  DelayLength=1  InitialCondition=boolean(0)
      settings: AttributesFormatString=%<InitialCondition>
  DelayEnable3 : hcu_lib/Basic_Blocks/DelayEnable
  Detect Increase6 : simulink/Logic and Bit Operations/Detect Increase  vinit=boolean(0)  OutDataTypeStr=boolean
  Equal36 : RelationalOperator  Operator=~=  OutDataTypeStr=boolean  RndMeth=Simplest
  Equal37 : RelationalOperator  Operator=>  OutDataTypeStr=boolean  RndMeth=Simplest
  Equal38 : RelationalOperator  Operator=<=  OutDataTypeStr=boolean  RndMeth=Simplest
  Equal39 : RelationalOperator  OutDataTypeStr=boolean  RndMeth=Simplest
  Equal41 : RelationalOperator  Operator===  OutDataTypeStr=boolean  RndMeth=Simplest
  Equal42 : RelationalOperator  Operator===  OutDataTypeStr=boolean  RndMeth=Simplest
  Equal43 : RelationalOperator  Operator=~=  OutDataTypeStr=boolean  RndMeth=Simplest
  Equal44 : RelationalOperator  Operator=~=  OutDataTypeStr=boolean  RndMeth=Simplest
  Logical Operator20 : Logic  Operator=OR  Inputs=5  AllPortsSameDT=off  OutDataTypeStr=boolean
  NOT3 : Logic  Operator=NOT  AllPortsSameDT=off  OutDataTypeStr=boolean
  OR2 : Logic  AllPortsSameDT=off  OutDataTypeStr=boolean
  OR3 : Logic  AllPortsSameDT=off  OutDataTypeStr=boolean
  OR5 : Logic  Operator=OR  AllPortsSameDT=off  OutDataTypeStr=boolean
  Relational Operator6 : RelationalOperator  Operator=<=  OutDataTypeStr=boolean  RndMeth=Simplest
  Relational Operator8 : RelationalOperator  Operator=<=  OutDataTypeStr=boolean  RndMeth=Simplest
  SR_Latch8 : hcu_lib/Basic_Blocks/SR_Latch
  VTQD_RegenLimIndSta_flg : Outport
  wires:
  [VTQD_RegenLimIndSta_flg] -> VTQD_RegenLimIndSta_flg/1
  BSCPIn_outputs/1 -> Bus Selector/1
  BInpConvert_outputs/1 -> Bus Selector1/1
  Bus Selector/1 -> [task_time_s]  "<task_time_s>"
  Bus Selector/2 -> [VTQD_RDCActive_enum]  "<VTQD_RDCActive_enum>"
  Bus Selector/3 -> [VINP_HVBattSOCDis_pct]  "<VINP_HVBattSOCDis_pct>"
  Bus Selector/4 -> [VINP_HVBMTempMin_C]  "<VINP_HVBMTempMin_C>"
  Bus Selector/5 -> [VINP_HVBMTempMax_C]  "<VINP_HVBMTempMax_C>"
  Bus Selector/6 -> [VPMM_DrivetrainSelect_enum]  "<VPMM_DrivetrainSelect_enum>"
  Bus Selector1/1 -> [VTQD_GearActualPosn_enum]  "<VTQD_GearActualPosn_enum>"
  BMain_outputs/1 -> Bus Selector2/1
  Bus Selector2/1 -> [VTQD_CoordWhlTqDemFr_Nm]  "<VTQD_CoordWhlTqDemFr_Nm>"
  Bus Selector2/2 -> [VTQD_CoordWhlTqDemRr_Nm]  "<VTQD_CoordWhlTqDemRr_Nm>"
  Bus Selector1/2 -> [VTQD_WhlTqCapGenFr_Nm]  "<VTQD_WhlTqCapGenFr_Nm>"
  [task_time_s] -> DelayEnable3/3
  OR5/1 -> Logical Operator20/5  "VTQD_RgnTqComLim_flg"
  Relational Operator8/1 -> OR3/2
  AND8/1 -> AND6/2
  [VTQD_RegenLimIndSta_flg] -> Delay17/1
  Delay17/1 -> DelayEnable3/1
  Logical Operator20/1 -> NOT3/1, Detect Increase6/1
  Constant91/1 -> Equal41/2
  NOT3/1 -> AND15/1
  [VTQD_CoordWhlTqDemFr_Nm] -> Relational Operator6/1
  Equal37/1 -> Logical Operator20/2
  Relational Operator6/1 -> OR2/2
  SR_Latch8/1 -> [VTQD_RegenLimIndSta_flg]  "VTQD_RegenLimIndSta_flg"
  Equal43/1 -> OR2/1
  OR2/1 -> OR5/1
  [VPMM_DrivetrainSelect_enum] -> Equal44/1
  OR3/1 -> OR5/2
  Constant95/1 -> Equal44/2
  Equal44/1 -> OR3/1
  [VTQD_WhlTqCapGenFr_Nm] -> Relational Operator6/2
  [VTQD_GearActualPosn_enum] -> Equal42/1
  [VPMM_DrivetrainSelect_enum] -> Equal43/1
  Constant94/1 -> Equal43/2
  Equal41/1 -> AND8/1
  [VTQD_GearActualPosn_enum] -> Equal41/1
  [VTQD_CoordWhlTqDemRr_Nm] -> Relational Operator8/1
  Constant126/1 -> DelayEnable3/2
  Constant92/1 -> Equal42/2
  [VINP_HVBMTempMax_C] -> Equal39/1
  Equal38/1 -> Logical Operator20/3
  Equal36/1 -> Logical Operator20/1
  Constant104/1 -> Equal39/2
  AND15/1 -> AND6/1
  Constant103/1 -> Equal38/2
  Equal39/1 -> Logical Operator20/4
  AND6/1 -> SR_Latch8/2
  [VINP_HVBattSOCDis_pct] -> Equal37/1
  [VTQD_RDCActive_enum] -> Equal36/1
  DelayEnable3/1 -> AND15/2
  Equal42/1 -> AND8/2
  [VINP_HVBMTempMin_C] -> Equal38/1
  Detect Increase6/1 -> SR_Latch8/1
  Constant106/1 -> Equal37/2
  Constant105/1 -> Equal36/2

== system tqdtqr_rebuild_V3/Output_Convert/SWC1 SWC2 set speed warning ==
  note: Merge warning
  note: SWC1 set speed warning
  note: SWC2 set speed warning
  BSCPIn_outputs : Inport
  BInpConvert_outputs : Inport  Port=2
  AND{,1,4,8} (4 alike) : Logic  AllPortsSameDT=off  OutDataTypeStr=boolean
  AND2 : Logic  Inputs=3  AllPortsSameDT=off  OutDataTypeStr=boolean
  AND3 : Logic  Operator=OR  AllPortsSameDT=off  OutDataTypeStr=boolean
  AND6 : Logic  Inputs=3  AllPortsSameDT=off  OutDataTypeStr=boolean
  AND7 : Logic  Operator=OR  AllPortsSameDT=off  OutDataTypeStr=boolean
  Bus Selector : BusSelector  OutputSignals=VINP_Distanceunit_flg,VVMC_MeterIndSpeed_raw32,VINP_SmartEcoModeSW_flg,VINP_SWCType_enum
  Bus Selector1 : BusSelector  OutputSignals=VTQD_SWC1SetSpd_kph,VTQD_SWCResUpSta_flg,VTQD_SWCSetdownSta_flg,VTQD_SWC2SetSpd_kph,VTQD_SWC2ScrollUpSta_flg,VTQD_SpdLim4SetSpd_raw32,VTQD_SWC2ResUpSta_flg,VTQD_SWC2SetdownSta_flg
  Constant{1,3,5,14,16,18} (6 alike) : Constant  Value=KTQD_SmartEcoLimitSpd_kph
  Constant{2,4,6,15,17,19} (6 alike) : Constant  Value=KTQD_SmartEcoLimitSpd_mph
  Constant77 : Constant  Value=ENUM_SWCTYPE_SWC
  Equal30 : RelationalOperator  Operator===  OutDataTypeStr=boolean  RndMeth=Simplest
  OR : Logic  Operator=OR  AllPortsSameDT=off  OutDataTypeStr=boolean
  OR1 : Logic  Operator=OR  AllPortsSameDT=off  OutDataTypeStr=boolean
  Relational Operator{,1..5} (6 alike) : RelationalOperator  OutDataTypeStr=boolean  RndMeth=Simplest
  Switch{,1..3,5..7} (7 alike) : Switch  Criteria=u2 ~= 0
      settings: AttributesFormatString=%<Criteria>
  VTQD_SetSpdLimWarn_flg : Outport
  wires:
  [VVMC_MeterIndSpeed_raw32] -> Relational Operator1/1
  Switch5/1 -> Relational Operator/2
  [VTQD_SWCResUpSta_flg] -> OR/1
  [VTQD_SWCResUpSta_flg] -> AND/2
  Switch7/1 -> Relational Operator2/2
  [VTQR_SWC1SetSpd_kph] -> Relational Operator/1
  AND7/1 -> AND8/1
  [VINP_Distanceunit_flg] -> Switch7/2
  AND6/1 -> AND7/2
  Constant18/1 -> Switch7/3
  Constant17/1 -> Switch6/1
  [VTQD_SWCSetDownSta_flg] -> OR/2
  Constant19/1 -> Switch7/1
  Switch6/1 -> Relational Operator1/2
  [VINP_SmartEcoModeSW_flg] -> AND8/2
  Relational Operator1/1 -> AND6/1
  Constant14/1 -> Switch5/3
  Constant15/1 -> Switch5/1
  [VINP_Distanceunit_flg] -> Switch6/2
  Constant16/1 -> Switch6/3
  Relational Operator2/1 -> AND6/3
  Relational Operator/1 -> AND/1
  [VTQR_SWC1SetSpd_kph] -> Relational Operator2/1
  [VINP_Distanceunit_flg] -> Switch5/2
  AND/1 -> AND7/1
  OR/1 -> AND6/2
  AND8/1 -> [VTQD_SWCSetSpdLimWarn_flg]  "VTQD_SetSpdLimWarn_flg"
  Relational Operator5/1 -> AND2/3
  AND1/1 -> AND3/1
  [VTQR_SWC2SetSpd_kph] -> Relational Operator3/1
  Constant4/1 -> Switch2/1
  Relational Operator4/1 -> AND2/1
  Constant6/1 -> Switch3/1
  AND3/1 -> AND4/1
  [VINP_Distanceunit_flg] -> Switch1/2
  [VTQD_SWC2ScrollUpSta_flg] -> AND1/2
  [VTQD_SWC2ResUpSta_flg] -> OR1/1
  [VTQD_SWC2SetDownSta_flg] -> OR1/2
  Switch2/1 -> Relational Operator4/2
  Switch3/1 -> Relational Operator5/2
  AND2/1 -> AND3/2
  Switch1/1 -> Relational Operator3/2
  Constant5/1 -> Switch3/3
  [VINP_SmartEcoModeSW_flg] -> AND4/2
  Constant2/1 -> Switch1/1
  [VINP_Distanceunit_flg] -> Switch2/2
  [VINP_Distanceunit_flg] -> Switch3/2
  Relational Operator3/1 -> AND1/1
  Constant3/1 -> Switch2/3
  [VTQD_SpdLim4SetSpd_raw32] -> Relational Operator4/1
  OR1/1 -> AND2/2
  [VTQR_SWC2SetSpd_kph] -> Relational Operator5/1
  Constant1/1 -> Switch1/3
  AND4/1 -> [VTQD_SWC2SetSpdLimWarn_flg]
  [VTQD_SetSpdLimWarn_flg] -> VTQD_SetSpdLimWarn_flg/1
  [VTQD_SWCSetSpdLimWarn_flg] -> Switch/1
  [VTQD_SWC2SetSpdLimWarn_flg] -> Switch/3
  Switch/1 -> [VTQD_SetSpdLimWarn_flg]  "VTQD_SetSpdLimWarn_flg"
  Equal30/1 -> Switch/2
  Constant77/1 -> Equal30/2
  [VINP_SWCType_enum] -> Equal30/1
  BSCPIn_outputs/1 -> Bus Selector/1
  BInpConvert_outputs/1 -> Bus Selector1/1
  Bus Selector1/1 -> [VTQR_SWC1SetSpd_kph]  "<VTQD_SWC1SetSpd_kph>"
  Bus Selector/1 -> [VINP_Distanceunit_flg]  "<VINP_Distanceunit_flg>"
  Bus Selector1/2 -> [VTQD_SWCResUpSta_flg]  "<VTQD_SWCResUpSta_flg>"
  Bus Selector/2 -> [VVMC_MeterIndSpeed_raw32]  "<VVMC_MeterIndSpeed_raw32>"
  Bus Selector1/3 -> [VTQD_SWCSetDownSta_flg]  "<VTQD_SWCSetdownSta_flg>"
  Bus Selector/3 -> [VINP_SmartEcoModeSW_flg]  "<VINP_SmartEcoModeSW_flg>"
  Bus Selector1/4 -> [VTQR_SWC2SetSpd_kph]  "<VTQD_SWC2SetSpd_kph>"
  Bus Selector1/5 -> [VTQD_SWC2ScrollUpSta_flg]  "<VTQD_SWC2ScrollUpSta_flg>"
  Bus Selector1/6 -> [VTQD_SpdLim4SetSpd_raw32]  "<VTQD_SpdLim4SetSpd_raw32>"
  Bus Selector1/7 -> [VTQD_SWC2ResUpSta_flg]  "<VTQD_SWC2ResUpSta_flg>"
  Bus Selector1/8 -> [VTQD_SWC2SetDownSta_flg]  "<VTQD_SWC2SetdownSta_flg>"
  Bus Selector/4 -> [VINP_SWCType_enum]  "<VINP_SWCType_enum>"
